simulink model "AL_model_YAW"  (R2023b)
settings: Solver=FixedStepAuto  StartTime=0.0  StopTime=t(end)  FixedStep=0.002  RelTol=1e-3
settings Model: Creator=franc  LastModifiedBy=franc

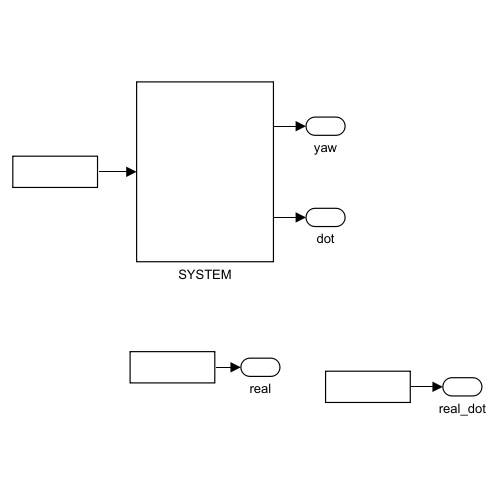
[thumbnail: Simulink's stored preview of the top-level diagram]
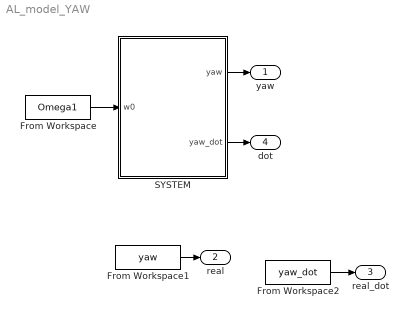
== system AL_model_YAW ==
  From Workspace : FromWorkspace  VariableName=Omega1
  From Workspace1 : FromWorkspace  VariableName=yaw
  From Workspace2 : FromWorkspace  VariableName=yaw_dot
  SYSTEM : Subsystem
  yaw : Outport
  real : Outport  Port=2
  real_dot : Outport  Port=3
  dot : Outport  Port=4
  wires:
  From Workspace/1 -> SYSTEM/1(w0)
  SYSTEM/1(yaw) -> yaw/1
  From Workspace1/1 -> real/1
  From Workspace2/1 -> real_dot/1
  SYSTEM/2(yaw_dot) -> dot/1

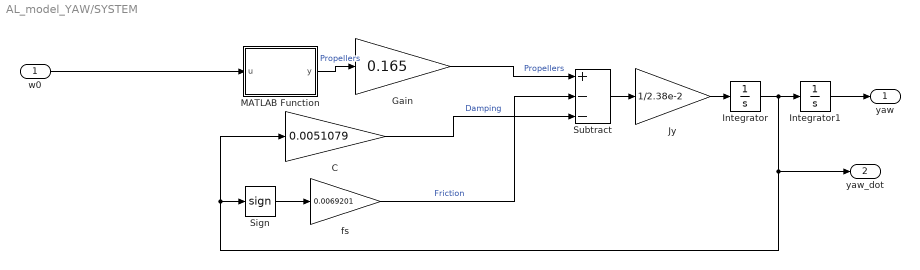
== system AL_model_YAW/SYSTEM ==
  w0 : Inport
  C : Gain  Gain=0.0051079
  Gain : Gain  Gain=0.165
  Integrator : Integrator
  Integrator1 : Integrator
  Jy : Gain  Gain=1/2.38e-2
  MATLAB Function : MATLAB Function  TreatAsAtomicUnit=on
  Sign : Signum
  Subtract : Sum  Inputs=+--
  fs : Gain  Gain=0.0069201
  yaw : Outport
  yaw_dot : Outport  Port=2
  wires:
  Jy/1 -> Integrator/1
  Gain/1 -> Subtract/1  "Propellers"
  Integrator1/1 -> yaw/1
  Integrator/1 -> Integrator1/1, yaw_dot/1, C/1, Sign/1
  Subtract/1 -> Jy/1
  C/1 -> Subtract/3  "Damping"
  Sign/1 -> fs/1
  w0/1 -> MATLAB Function/1(u)
  fs/1 -> Subtract/2  "Friction"
  MATLAB Function/1(y) -> Gain/1  "Propellers"

== matlab function AL_model_YAW/SYSTEM/MATLAB Function ==
  data: u input; y output
function y = fcn(u)
y = -2.522922e-05*u+4.01487e-06*u^2;
